simulink model "PMSMdq"  (R2024a)
settings: Solver=ode45  StartTime=0.0  StopTime=10  MaxStep=1  RelTol=1e-3  EnableMultiTasking=on
undefined symbols (not defined in the file or in its folder): Battery, Control, Environment, Motor, Vehicle
libraries: simulink x5, simulink_extras x4, SignalEditorBlockLib x2
settings Model: Creator=Daniel Montesinos  LastModifiedBy=citcea
settings SolverCC: AlgebraicLoopSolver=TrustRegion
settings DataIOCC: LimitDataPoints=on  SaveFormat=Array  SignalLoggingSaveFormat=ModelDataLogs  ReturnWorkspaceOutputs=off
settings OptimizationCC: ReuseModelBlockBuffer=off  ExpressionDepthLimit=2147483647  LifeSpan=inf
settings DebuggingCC: UnderspecifiedInitializationDetection=Classic  MergeDetectMultiDrivingBlocksExec=none  SolverPrmCheckMsg=warning  FcnCallInpInsideContextMsg=warning  UnconnectedInputMsg=warning  UnconnectedOutputMsg=warning  UnconnectedLineMsg=warning  AllowSymbolicDim=off  StateNameClashWarn=warning  SFUnexpectedBacktrackingDiag=warning  SFNoUnconditionalDefaultTransitionDiag=warning  SFExecutionAtInitializationDiag=none  ArithmeticOperatorsInVariantConditions=warning
settings HardwareCC: ProdBitPerPointer=32  ProdBitPerSizeT=32  ProdBitPerPtrDiffT=32  ProdLargestAtomicFloat=None  ProdIntDivRoundTo=Undefined  ProdEndianess=Unspecified  ProdWordSize=32  ProdHWDeviceType=32-bit Generic
settings ModelReferenceCC: EnableRefExpFcnMdlSchedulingChecks=on  PropagateSignalLabelsOutOfModel=off
settings SFSimCC: SimUseLocalCustomCode=off  CustomCodeUndefinedFunction=UseInterfaceOnly
settings RTWCC: RTWUseLocalCustomCode=off  GPUComputeCapability=3.5  DLArmComputeVersion=19.05
settings CodeAppCC: StateflowObjectComments=on
settings GRTTargetCC: TargetLangStandard=C89/C90 (ANSI)  CombineOutputUpdateFcns=off  GRTInterface=on
settings ConfigComp: CovMetricSettings=dw  CovSaveCumulativeToWorkspaceVar=on  CovSaveSingleToWorkspaceVar=on  CovExternalEMLEnable=off  CovSFcnEnable=off

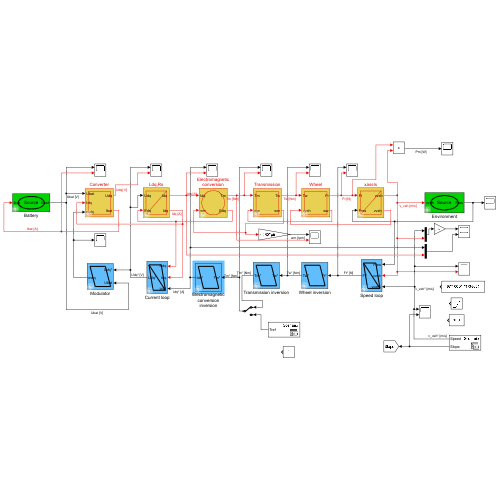
[thumbnail: Simulink's stored preview of the top-level diagram]
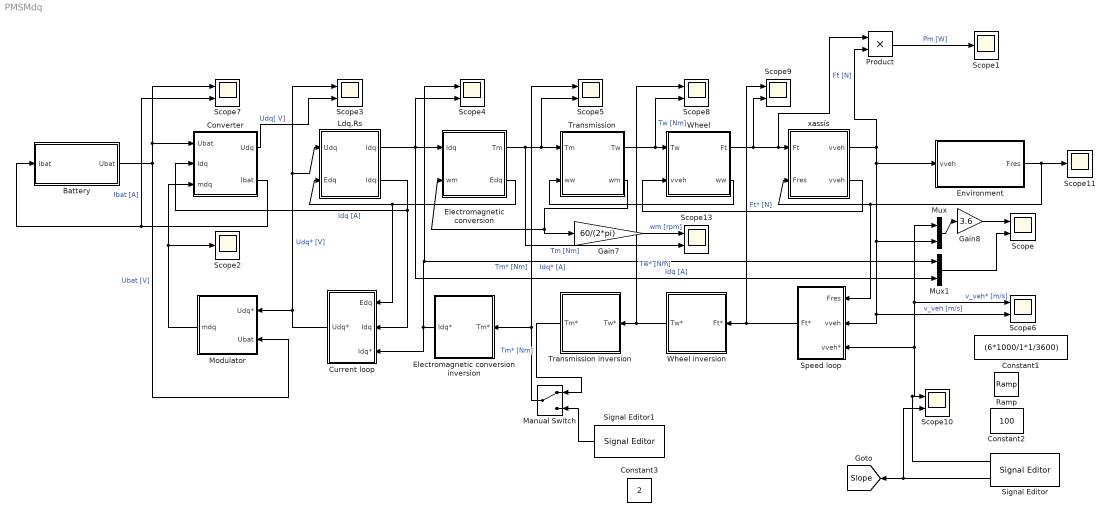
== system PMSMdq ==
  Battery : Subsystem  AncestorBlock=simulink/REM/SE
      mask Display:
      | plot(0,0,100,100, 1.2*[50,57.68,60.77,63.08,64.97,66.58,68,69.26,70.4, 	71.42,72.36,78.28,80,78.28,72.36,71.42,70.4, 	69.26,68,66.58,64.97,63.08,60.77,57.68,50,42.32, 	39.23,36.92,35.03,33.42,32,30.74,29.6,28.58, 	27.64,21.72,20,21.72,27.64,28.58,29.6,30.74,32, 	33.42,35.03,36.92,39.23,42.32,50]-10, 1.2*[20,21,22,23,24,25,26,27,28,29,30,40,50,60,70,71,72, 	73,74,75,76,77,78,79,80,79,78,77,76,75,74,73,72, 	71,70,60,50,40,30,29,28,27,26,25,24,23,22,21,20]-10)
      | disp('Source')
  Constant1 : Constant  Value=(6*1000/1*1/3600)
  Constant2 : Constant  Value=100
  Constant3 : Constant  Value=2
  Converter : Subsystem  AncestorBlock=simulink/REM/EC Elec  mask(Hacheur){}
      mask Display: plot(0,0,100,100,[10,10,90,90,10],[90,10,10,90,90])
  Current loop : Subsystem  AncestorBlock=simulink/SMC/Asservissement Correcteur IP
      mask Display: plot(0,0,100,100, [10,30,90,70,10,90],[90,10,10,90,90,10])
  Electromagnetic conversion : Subsystem  AncestorBlock=simulink/REM/EC EM
      mask Display: plot(0,0,100,100, 1.4*[50,57.68,60.77,63.08,64.97,66.58,68,69.26,70.4, 	71.42,72.36,78.28,80,78.28,72.36,71.42,70.4, 	69.26,68,66.58,64.97,63.08,60.77,57.68,50,42.32, 	39.23,36.92,35.03,33.42,32,30.74,29.6,28.58, 	27.64,21.72,20,21.72,27.64,28.58,29.6,30.74,32, 	33.42,35.03,36.92,39.23,42.32,50]-20, 1.4*[20,21,22,23,24,25,26,27,28,29,30,40,50,60,70,71,72, 	73,74,75,76,77,78,79,80,79,78,77,76,75,74,73,72, 	71,70,60,50,40,30,29,28,27,26,25,24,23,22,21,20]-20)
  Electromagnetic conversion inversion : Subsystem  AncestorBlock=simulink/SMC/Inversion EC avec mesure
      mask Display: plot(0,0,100,100,[10,30,90,70,10],[90,10,10,90,90])
  Environment : Subsystem  AncestorBlock=simulink/REM/SE
      mask Display:
      | plot(0,0,100,100, 1.2*[50,57.68,60.77,63.08,64.97,66.58,68,69.26,70.4, 	71.42,72.36,78.28,80,78.28,72.36,71.42,70.4, 	69.26,68,66.58,64.97,63.08,60.77,57.68,50,42.32, 	39.23,36.92,35.03,33.42,32,30.74,29.6,28.58, 	27.64,21.72,20,21.72,27.64,28.58,29.6,30.74,32, 	33.42,35.03,36.92,39.23,42.32,50]-10, 1.2*[20,21,22,23,24,25,26,27,28,29,30,40,50,60,70,71,72, 	73,74,75,76,77,78,79,80,79,78,77,76,75,74,73,72, 	71,70,60,50,40,30,29,28,27,26,25,24,23,22,21,20]-10)
      | disp('Source')
  Gain7 : Gain  Gain=60/(2*pi)
  Gain8 : Gain  Gain=3.6
  Ldq,Rs : Subsystem  AncestorBlock=simulink/REM/EA  mask(CM){}
      mask Display: plot(0,0,100,100,[10,10,90,90,10],[90,10,10,90,90], [10,90],[10,90])
  Manual Switch : ManualSwitch
  Modulator : Subsystem  AncestorBlock=simulink/SMC/Inversion EC avec mesure
      mask Display: plot(0,0,100,100,[10,30,90,70,10],[90,10,10,90,90])
  Mux : Mux  Inputs=2
  Mux1 : Mux  Inputs=2
  Product : Product
  Ramp : simulink/Sources/Ramp  slope=(3*1000/1*1/3600)/2  start=0  InitialOutput=0
  Scope{,3..10,13} (10 alike) : Scope  NumInputPorts=2
  Scope1 : Scope
  Scope11 : Scope
  Scope2 : Scope
  Signal Editor : SignalEditorBlockLib/Signal Editor  FileName=SpeedRef.mat  ActiveScenario=Scenario  ActiveSignal=Speed  IsBus=off  OutputBusObjectStr=Bus: BusObject  SampleTime=0  Interpolate=off  ZeroCross=off  OutputAfterFinalValue=Setting to zero  Unit=inherit  PreserveSignalName=on  ApplySigPropsToAllScenarios=on  ApplySigPropsToAllSignals=off
  Signal Editor1 : SignalEditorBlockLib/Signal Editor  FileName=Tref.mat  ActiveScenario=Scenario  ActiveSignal=Tref  IsBus=off  OutputBusObjectStr=Bus: BusObject  SampleTime=0  Interpolate=off  ZeroCross=off  OutputAfterFinalValue=Setting to zero  Unit=inherit  PreserveSignalName=on  ApplySigPropsToAllScenarios=on  ApplySigPropsToAllSignals=off
  Speed loop : Subsystem  AncestorBlock=simulink/SMC/Asservissement Correcteur IP
      mask Display: plot(0,0,100,100, [10,30,90,70,10,90],[90,10,10,90,90,10])
  Transmission : Subsystem  AncestorBlock=simulink/REM/EC Elec  mask(Hacheur){}
      mask Display: plot(0,0,100,100,[10,10,90,90,10],[90,10,10,90,90])
  Transmission inversion : Subsystem  AncestorBlock=simulink/SMC/Inversion EC avec mesure
      mask Display: plot(0,0,100,100,[10,30,90,70,10],[90,10,10,90,90])
  Wheel : Subsystem  AncestorBlock=simulink/REM/EC Elec  mask(Hacheur){}
      mask Display: plot(0,0,100,100,[10,10,90,90,10],[90,10,10,90,90])
  Wheel inversion : Subsystem  AncestorBlock=simulink/SMC/Inversion EC avec mesure
      mask Display: plot(0,0,100,100,[10,30,90,70,10],[90,10,10,90,90])
  xassís : Subsystem  AncestorBlock=simulink/REM/EA  mask(CM){}
      mask Display: plot(0,0,100,100,[10,10,90,90,10],[90,10,10,90,90], [10,90],[10,90])
  tag scope: Slope=global
  wires:
  xassís/1(vveh) -> Product/2, Environment/1(vveh), Scope6/2, Speed loop/2(vveh), Mux/2  "v_veh [m/s]"
  Environment/1(Fres) -> Scope11/1, Speed loop/1(Fres), xassís/2(Fres)
  Mux/1 -> Gain8/1
  xassís/2("vveh ") -> Wheel/2(vveh)
  Transmission/1(Tw) -> Scope8/2, Wheel/1(Tw)  "Tw [Nm]"
  Wheel/2(ww) -> Transmission/2(ww)
  Wheel inversion/1(Tw*) -> Scope8/1, Transmission inversion/1(Tw*)  "Tw* [Nm]"
  Transmission/2(wm) -> Electromagnetic conversion/2(wm), Gain7/1
  Electromagnetic conversion/1(Tm) -> Scope13/2, Scope5/2, Transmission/1(Tm)  "Tm [Nm]"
  Ldq,Rs/1("Idq ") -> Scope4/2, Electromagnetic conversion/1(Idq), Mux1/2  "Idq [A]"
  Electromagnetic conversion/2(Edq) -> Current loop/1(Edq), Ldq,Rs/2(Edq)
  Electromagnetic conversion inversion/1(Idq*) -> Scope4/1, Mux1/1, Current loop/3(Idq*)  "Idq* [A]"
  Ldq,Rs/2(Idq) -> Current loop/2(Idq), Converter/2(Idq)  "Idq [A]"
  Manual Switch/1 -> Scope5/1, Electromagnetic conversion inversion/1(Tm*)  "Tm* [Nm]"
  Modulator/1(mdq) -> Converter/3(mdq), Scope2/1
  Converter/2(Ibat) -> Battery/1(Ibat), Scope7/2  "Ibat [A]"
  Battery/1(Ubat) -> Modulator/2(Ubat), Converter/1(Ubat), Scope7/1  "Ubat [V]"
  Speed loop/1(Ft*) -> Scope9/1, Wheel inversion/1(Ft*)  "Ft* [N]"
  Wheel/1(Ft) -> Scope9/2, Product/1, xassís/1(Ft)  "Ft [N]"
  Current loop/1(Udq*) -> Ldq,Rs/1(Udq), Scope3/1, Modulator/1(Udq*)  "Udq* [V]"
  Converter/1(Udq) -> Scope3/2  "Udq[ V]"
  Gain7/1 -> Scope13/1  "wm [rpm]"
  Gain8/1 -> Scope/1
  Mux1/1 -> Scope/2
  Signal Editor/1 -> Speed loop/3(vveh*), Scope6/1, Mux/1, Scope10/1  "v_veh* [m/s]"
  Product/1 -> Scope1/1  "Pm [W]"
  Signal Editor/2 -> Scope10/2, [Slope]
  Signal Editor1/1 -> Manual Switch/2
  Transmission inversion/1(Tm*) -> Manual Switch/1  "Tm* [Nm]"

== system PMSMdq/Battery ==
  Ibat : Inport
  Constant : Constant  Value=Battery.Electrical.Ubat
  Terminator : Terminator
  Ubat : Outport  InitialOutput=0  VectorParamsAs1DForOutWhenUnconnected=off
  wires:
  Ibat/1 -> Terminator/1
  Constant/1 -> Ubat/1

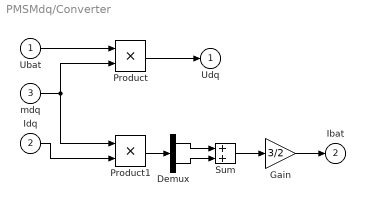
== system PMSMdq/Converter ==
  Ubat : Inport
  Idq : Inport  Port=2
  mdq : Inport  Port=3
  Demux : Demux  Outputs=2
  Gain : Gain  Gain=3/2
  Product : Product
  Product1 : Product
  Sum : Sum
  Udq : Outport  InitialOutput=0  VectorParamsAs1DForOutWhenUnconnected=off
  Ibat : Outport  Port=2  InitialOutput=0  VectorParamsAs1DForOutWhenUnconnected=off
  wires:
  Ubat/1 -> Product/1
  mdq/1 -> Product1/1, Product/2
  Product/1 -> Udq/1
  Product1/1 -> Demux/1
  Demux/1 -> Sum/1
  Demux/2 -> Sum/2
  Sum/1 -> Gain/1
  Gain/1 -> Ibat/1
  Idq/1 -> Product1/2

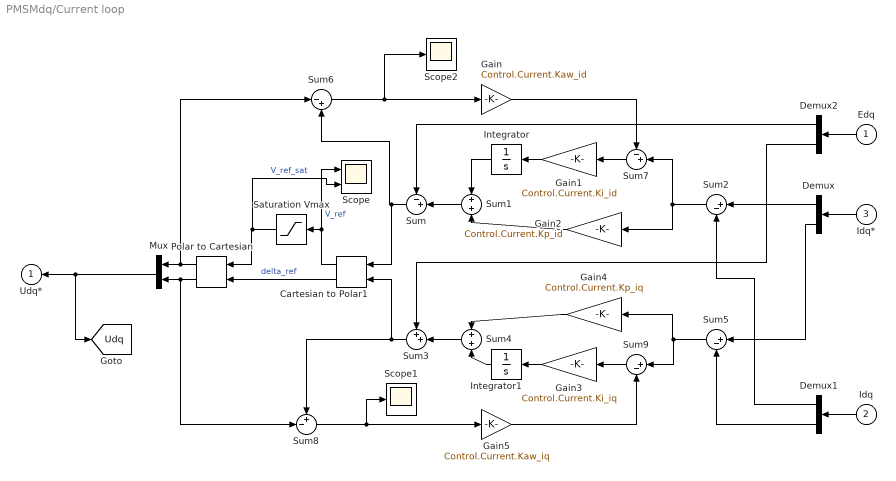
== system PMSMdq/Current loop ==
  Edq : Inport
  Idq : Inport  Port=2
  Idq* : Inport  Port=3
  Cartesian to Polar1 : simulink_extras/Transformations/Cartesian to Polar
  Demux : Demux  Outputs=2
  Demux1 : Demux  Outputs=2
  Demux2 : Demux  Outputs=2
  Gain : Gain  Gain=Control.Current.Kaw_id
  Gain1 : Gain  Gain=Control.Current.Ki_id
  Gain2 : Gain  Gain=Control.Current.Kp_id
  Gain3 : Gain  Gain=Control.Current.Ki_iq
  Gain4 : Gain  Gain=Control.Current.Kp_iq
  Gain5 : Gain  Gain=Control.Current.Kaw_iq
  Integrator : Integrator
  Integrator1 : Integrator
  Mux : Mux  Inputs=2
  Polar to Cartesian : simulink_extras/Transformations/Polar to Cartesian
  Saturation Vmax : Saturate  UpperLimit=Motor.Electrical.Umax  LowerLimit=-Motor.Electrical.Umax
  Scope : Scope  NumInputPorts=2
  Scope1 : Scope
  Scope2 : Scope
  Sum : Sum  Inputs=-+|
  Sum1 : Sum
  Sum2 : Sum  Inputs=|+-
  Sum3 : Sum  Inputs=++|
  Sum4 : Sum
  Sum5 : Sum  Inputs=|+-
  Sum6 : Sum  Inputs=|-+
  Sum7 : Sum  Inputs=-+|
  Sum8 : Sum  Inputs=+-|
  Sum9 : Sum  Inputs=|+-
  Udq* : Outport  InitialOutput=0  VectorParamsAs1DForOutWhenUnconnected=off
  tag scope: Udq=global
  wires:
  Sum1/1 -> Sum/2
  Gain1/1 -> Integrator/1
  Sum2/1 -> Sum7/2, Gain2/1
  Integrator1/1 -> Sum4/2
  Gain3/1 -> Integrator1/1
  Gain4/1 -> Sum4/1
  Sum5/1 -> Sum9/1, Gain4/1
  Sum4/1 -> Sum3/2
  Idq*/1 -> Demux/1
  Demux/1 -> Sum2/1
  Demux/2 -> Sum5/1
  Idq/1 -> Demux1/1
  Demux1/1 -> Sum2/2
  Demux1/2 -> Sum5/2
  Edq/1 -> Demux2/1
  Demux2/2 -> Sum3/1
  Mux/1 -> [Udq], Udq*/1
  Demux2/1 -> Sum/1
  Cartesian to Polar1/1 -> Scope/1, Saturation Vmax/1  "V_ref"
  Saturation Vmax/1 -> Scope/2, Polar to Cartesian/1  "V_ref_sat"
  Cartesian to Polar1/2 -> Polar to Cartesian/2  "delta_ref"
  Sum/1 -> Sum6/2, Cartesian to Polar1/1
  Sum3/1 -> Sum8/1, Cartesian to Polar1/2
  Polar to Cartesian/1 -> Sum6/1, Mux/1
  Polar to Cartesian/2 -> Sum8/2, Mux/2
  Integrator/1 -> Sum1/1
  Gain2/1 -> Sum1/2
  Sum7/1 -> Gain1/1
  Sum6/1 -> Scope2/1, Gain/1
  Gain/1 -> Sum7/1
  Sum9/1 -> Gain3/1
  Sum8/1 -> Scope1/1, Gain5/1
  Gain5/1 -> Sum9/2

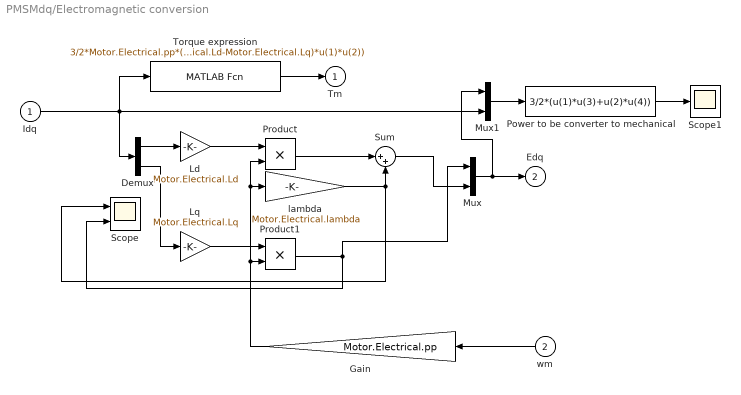
== system PMSMdq/Electromagnetic conversion ==
  Idq : Inport
  wm : Inport  Port=2
  Demux : Demux  Outputs=2
  Gain : Gain  Gain=Motor.Electrical.pp
  Ld : Gain  Gain=Motor.Electrical.Ld
  Lq : Gain  Gain=Motor.Electrical.Lq
  Mux : Mux  Inputs=2
  Mux1 : Mux  Inputs=2
  Power to be converter to mechanical : MATLABFcn  MATLABFcn=3/2*(u(1)*u(3)+u(2)*u(4))
  Product : Product
  Product1 : Product
  Scope : Scope  NumInputPorts=2
  Scope1 : Scope
  Sum : Sum  Inputs=|++
  Torque expression : MATLABFcn  MATLABFcn=3/2*Motor.Electrical.pp*(Motor.Electrical.lambda*u(2)+(Motor.Electrical.Ld-Motor.Electrical.Lq)*u(1)*u(2))  OutputDimensions=1
  lambda : Gain  Gain=Motor.Electrical.lambda
  Tm : Outport  InitialOutput=0  VectorParamsAs1DForOutWhenUnconnected=off
  Edq : Outport  Port=2  InitialOutput=0  VectorParamsAs1DForOutWhenUnconnected=off
  wires:
  Torque expression/1 -> Tm/1
  Idq/1 -> Demux/1, Torque expression/1, Mux1/2
  Demux/1 -> Ld/1
  Demux/2 -> Lq/1
  Ld/1 -> Product/1
  wm/1 -> Gain/1
  Lq/1 -> Product1/1
  Product/1 -> Sum/1
  lambda/1 -> Scope/1, Sum/2
  Product1/1 -> Scope/2, Mux/1
  Mux/1 -> Mux1/1, Edq/1
  Mux1/1 -> Power to be converter to mechanical/1
  Power to be converter to mechanical/1 -> Scope1/1
  Sum/1 -> Mux/2
  Gain/1 -> Product/2, lambda/1, Product1/2

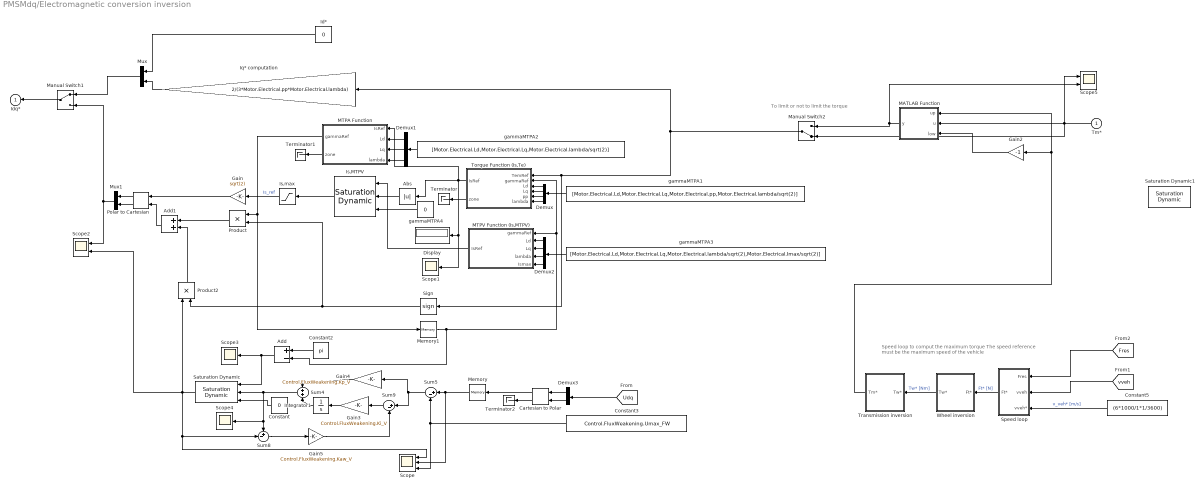
== system PMSMdq/Electromagnetic conversion inversion ==
  note: To limit or not to limit the torque
  note: Speed loop to comput the maximum torque
      | The speed reference must be the maximum speed of the vehicle
  Tm* : Inport
  Abs : Abs  SaturateOnIntegerOverflow=off
  Add : Sum  Inputs=+-
  Add1 : Sum
  Cartesian to Polar : simulink_extras/Transformations/Cartesian to Polar
  Constant : Constant  Value=0
  Constant2 : Constant  Value=pi
  Constant3 : Constant  Value=Control.FluxWeakening.Umax_FW  SampleTime=-1
  Constant5 : Constant  Value=(6*1000/1*1/3600)
  Demux : Demux
  Demux1 : Demux  Outputs=3
  Demux2 : Demux
  Demux3 : Demux  Outputs=2
  Display : Display
  Gain : Gain  Gain=sqrt(2)
  Gain2 : Gain  Gain=-1
  Gain3 : Gain  Gain=Control.FluxWeakening.Ki_V
  Gain4 : Gain  Gain=Control.FluxWeakening.Kp_V
  Gain5 : Gain  Gain=Control.FluxWeakening.Kaw_V
  Id* : Constant  Value=0
  Integrator1 : Integrator
  Iq* computation : Gain  Gain=2/(3*Motor.Electrical.pp*Motor.Electrical.lambda)
  Is,MTPV : simulink/Discontinuities/Saturation Dynamic  OutMin=[]  OutMax=[]  OutDataTypeStr=Inherit: Same as second input  OutDataType=fixdt(1, 16)  OutScaling=2^-10  DoSatur=off
  Is,max : Saturate  UpperLimit=Motor.Electrical.Imax  LowerLimit=0
  MATLAB Function : MATLAB Function  TreatAsAtomicUnit=on
  MTPA Function : MATLAB Function  TreatAsAtomicUnit=on
  MTPV Function (Is,MTPV) : MATLAB Function  TreatAsAtomicUnit=on
  Manual Switch1 : ManualSwitch
  Manual Switch2 : ManualSwitch  CurrentSetting=0
  Memory : Memory
  Memory1 : Memory  InitialCondition=pi/2
  Mux : Mux  Inputs=2
  Mux1 : Mux  Inputs=2
  Polar to Cartesian : simulink_extras/Transformations/Polar to Cartesian
  Product : Product
  Product2 : Product
  Saturation Dynamic : simulink/Discontinuities/Saturation Dynamic  OutMin=[]  OutMax=[]  OutDataTypeStr=Inherit: Same as second input  OutDataType=fixdt(1, 16)  OutScaling=2^-10  DoSatur=off
  Saturation Dynamic1 : simulink/Discontinuities/Saturation Dynamic  OutMin=[]  OutMax=[]  OutDataTypeStr=Inherit: Same as second input  OutDataType=fixdt(1, 16)  OutScaling=2^-10  DoSatur=off
  Scope : Scope  NumInputPorts=3
  Scope1 : Scope
  Scope2 : Scope  NumInputPorts=2
  Scope3 : Scope
  Scope4 : Scope
  Scope5 : Scope  NumInputPorts=2
  Sign : Signum
  Speed loop : Subsystem  AncestorBlock=simulink/SMC/Asservissement Correcteur IP
      mask Display: plot(0,0,100,100, [10,30,90,70,10,90],[90,10,10,90,90,10])
  Sum4 : Sum
  Sum5 : Sum  Inputs=|+-
  Sum8 : Sum  Inputs=+-|
  Sum9 : Sum  Inputs=|+-
  Terminator : Terminator
  Terminator1 : Terminator
  Terminator2 : Terminator
  Torque Function (Is,Te) : MATLAB Function  TreatAsAtomicUnit=on
  Transmission inversion : Subsystem  AncestorBlock=simulink/SMC/Inversion EC avec mesure
      mask Display: plot(0,0,100,100,[10,30,90,70,10],[90,10,10,90,90])
  Wheel inversion : Subsystem  AncestorBlock=simulink/SMC/Inversion EC avec mesure
      mask Display: plot(0,0,100,100,[10,30,90,70,10],[90,10,10,90,90])
  gammaMTPA1 : Constant  Value=[Motor.Electrical.Ld,Motor.Electrical.Lq,Motor.Electrical.pp,Motor.Electrical.lambda/sqrt(2)]  SampleTime=-1
  gammaMTPA2 : Constant  Value=[Motor.Electrical.Ld,Motor.Electrical.Lq,Motor.Electrical.lambda/sqrt(2)]  SampleTime=-1
  gammaMTPA3 : Constant  Value=[Motor.Electrical.Ld,Motor.Electrical.Lq,Motor.Electrical.lambda/sqrt(2),Motor.Electrical.Imax/sqrt(2)]  SampleTime=-1
  gammaMTPA4 : Constant  Value=0  SampleTime=-1
  Idq* : Outport  InitialOutput=0  VectorParamsAs1DForOutWhenUnconnected=off
  wires:
  MATLAB Function/1(y) -> Scope5/2, Manual Switch2/1
  gammaMTPA1/1 -> Demux/1
  Demux1/1 -> MTPA Function/2(Ld)
  Torque Function (Is,Te)/1(IsRef) -> Scope1/1, Display/1, Abs/1, MTPA Function/1(IsRef)
  MTPV Function (Is,MTPV)/1(IsRef) -> Is,MTPV/1
  gammaMTPA2/1 -> Demux1/1
  Demux2/2 -> MTPV Function (Is,MTPV)/3(Lq)
  Demux/1 -> Torque Function (Is,Te)/3(Ld)
  Demux1/3 -> MTPA Function/4(lambda)
  Demux2/4 -> MTPV Function (Is,MTPV)/5(Ismax)
  Demux/3 -> Torque Function (Is,Te)/5(pp)
  Demux/4 -> Torque Function (Is,Te)/6(lambda)
  Demux/2 -> Torque Function (Is,Te)/4(Lq)
  gammaMTPA3/1 -> Demux2/1
  MTPA Function/2(zone) -> Terminator1/1
  Is,MTPV/1 -> Is,max/1
  Torque Function (Is,Te)/2(zone) -> Terminator/1
  Demux1/2 -> MTPA Function/3(Lq)
  gammaMTPA4/1 -> Is,MTPV/3
  Demux2/3 -> MTPV Function (Is,MTPV)/4(lambda)
  Demux2/1 -> MTPV Function (Is,MTPV)/2(Ld)
  Is,max/1 -> Gain/1  "Is_ref"
  MTPA Function/1(gammaRef) -> Memory1/1, Product/1
  Memory1/1 -> Add/2, MTPV Function (Is,MTPV)/1(gammaRef), Torque Function (Is,Te)/2(gammaRef)
  Polar to Cartesian/1 -> Mux1/1
  Polar to Cartesian/2 -> Mux1/2
  Mux1/1 -> Scope2/1, Manual Switch1/2
  Gain/1 -> Polar to Cartesian/1
  Abs/1 -> Is,MTPV/2
  Sign/1 -> Product2/2, Product/2
  Demux3/2 -> Cartesian to Polar/2
  Demux3/1 -> Cartesian to Polar/1
  [Udq] -> Demux3/1
  Gain5/1 -> Sum9/2
  Cartesian to Polar/1 -> Memory/1
  Sum5/1 -> Gain4/1, Sum9/1
  Sum4/1 -> Scope4/1, Sum8/1, Saturation Dynamic/2
  Gain3/1 -> Integrator1/1
  Gain4/1 -> Sum4/1
  Constant3/1 -> Sum5/2, Scope/3
  Sum9/1 -> Gain3/1
  Integrator1/1 -> Sum4/2
  Cartesian to Polar/2 -> Terminator2/1
  Constant/1 -> Saturation Dynamic/3
  Add/1 -> Scope3/1, Saturation Dynamic/1
  Constant2/1 -> Add/1
  Sum8/1 -> Gain5/1
  Saturation Dynamic/1 -> Scope/1, Sum8/2, Scope2/2, Product2/1
  Product/1 -> Add1/1
  Add1/1 -> Polar to Cartesian/2
  Product2/1 -> Add1/2
  Memory/1 -> Scope/2, Sum5/1
  Manual Switch1/1 -> Idq*/1
  Mux/1 -> Manual Switch1/1
  Iq* computation/1 -> Mux/2
  Id*/1 -> Mux/1
  Transmission inversion/1(Tm*) -> MATLAB Function/1(up), Gain2/1
  Gain2/1 -> MATLAB Function/3(low)
  Tm*/1 -> MATLAB Function/2(u), Manual Switch2/2, Scope5/1
  Manual Switch2/1 -> Iq* computation/1, Sign/1, Torque Function (Is,Te)/1(TemRef)
  Constant5/1 -> Speed loop/3(vveh*)  "v_veh* [m/s]"
  Speed loop/1(Ft*) -> Wheel inversion/1(Ft*)  "Ft* [N]"
  Wheel inversion/1(Tw*) -> Transmission inversion/1(Tw*)  "Tw* [Nm]"
  [vveh] -> Speed loop/2(vveh)
  [Fres] -> Speed loop/1(Fres)

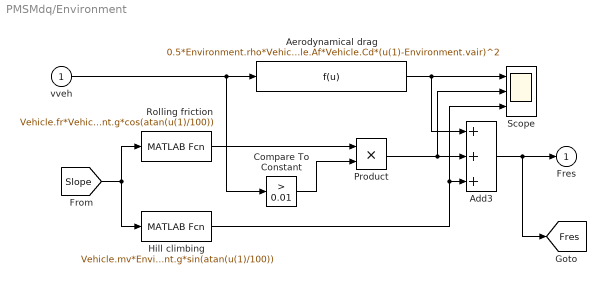
== system PMSMdq/Environment ==
  vveh : Inport
  Add3 : Sum  Inputs=+++
  Aerodynamical drag : Fcn  Expr=0.5*Environment.rho*Vehicle.Af*Vehicle.Cd*(u(1)-Environment.vair)^2
  Compare To Constant : simulink/Logic and Bit Operations/Compare To Constant  relop=>  const=0.01  OutDataTypeStr=boolean  ZeroCross=off
  Hill climbing : MATLABFcn  MATLABFcn=Vehicle.mv*Environment.g*sin(atan(u(1)/100))
  Product : Product
  Rolling friction : MATLABFcn  MATLABFcn=Vehicle.fr*Vehicle.mv*Environment.g*cos(atan(u(1)/100))
  Scope : Scope  NumInputPorts=3
  Fres : Outport  InitialOutput=0  VectorParamsAs1DForOutWhenUnconnected=off
  tag scope: Fres=global
  wires:
  Aerodynamical drag/1 -> Scope/1, Add3/1
  Hill climbing/1 -> Scope/3, Add3/3
  Product/1 -> Scope/2, Add3/2
  Add3/1 -> [Fres], Fres/1
  vveh/1 -> Compare To Constant/1, Aerodynamical drag/1
  Compare To Constant/1 -> Product/2
  Rolling friction/1 -> Product/1
  [Slope] -> Hill climbing/1, Rolling friction/1

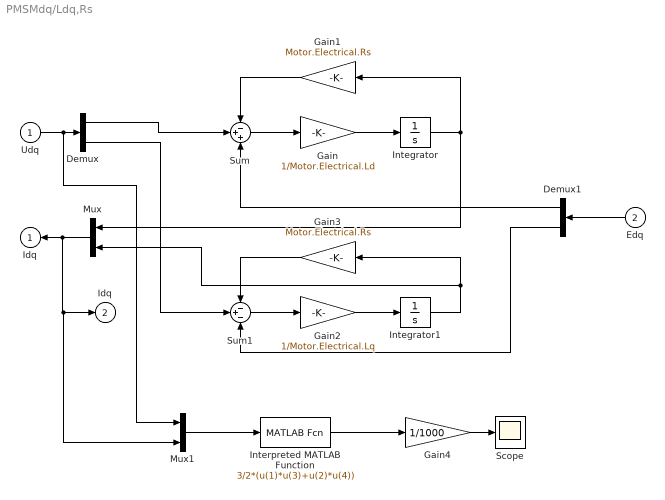
== system PMSMdq/Ldq,Rs ==
  Udq : Inport
  Edq : Inport  Port=2
  Demux : Demux  Outputs=2
  Demux1 : Demux  Outputs=2
  Gain : Gain  Gain=1/Motor.Electrical.Ld
  Gain1 : Gain  Gain=Motor.Electrical.Rs
  Gain2 : Gain  Gain=1/Motor.Electrical.Lq
  Gain3 : Gain  Gain=Motor.Electrical.Rs
  Gain4 : Gain  Gain=1/1000
  Integrator : Integrator
  Integrator1 : Integrator
  Interpreted MATLAB Function : MATLABFcn  MATLABFcn=3/2*(u(1)*u(3)+u(2)*u(4))
  Mux : Mux  Inputs=2
  Mux1 : Mux  Inputs=2
  Scope : Scope
  Sum : Sum  Inputs=-++
  Sum1 : Sum  Inputs=-+-
  "Idq " : Outport  InitialOutput=0  VectorParamsAs1DForOutWhenUnconnected=off
  Idq : Outport  Port=2  InitialOutput=0  VectorParamsAs1DForOutWhenUnconnected=off
  wires:
  Integrator/1 -> Mux/1, Gain1/1
  Gain/1 -> Integrator/1
  Sum/1 -> Gain/1
  Gain1/1 -> Sum/1
  Gain3/1 -> Sum1/1
  Gain2/1 -> Integrator1/1
  Integrator1/1 -> Gain3/1, Mux/2
  Sum1/1 -> Gain2/1
  Udq/1 -> Mux1/1, Demux/1
  Demux/1 -> Sum/2
  Demux/2 -> Sum1/2
  Mux/1 -> Mux1/2, Idq/1, "Idq "/1
  Edq/1 -> Demux1/1
  Mux1/1 -> Interpreted MATLAB Function/1
  Interpreted MATLAB Function/1 -> Gain4/1
  Gain4/1 -> Scope/1
  Demux1/1 -> Sum/3
  Demux1/2 -> Sum1/3

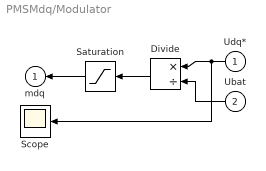
== system PMSMdq/Modulator ==
  Udq* : Inport
  Ubat : Inport  Port=2
  Divide : Product  Inputs=*/
  Saturation : Saturate  UpperLimit=1  LowerLimit=-1
  Scope : Scope
  mdq : Outport  InitialOutput=0  VectorParamsAs1DForOutWhenUnconnected=off
  wires:
  Udq*/1 -> Scope/1, Divide/1
  Ubat/1 -> Divide/2
  Divide/1 -> Saturation/1
  Saturation/1 -> mdq/1

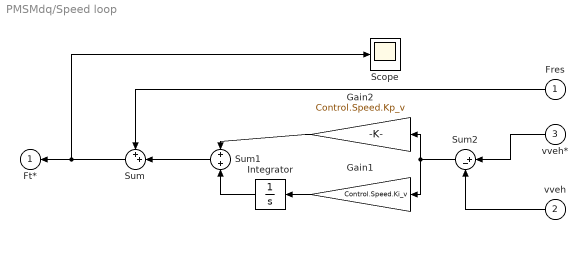
== system PMSMdq/Speed loop ==
  Fres : Inport
  vveh : Inport  Port=2
  vveh* : Inport  Port=3
  Gain1 : Gain  Gain=Control.Speed.Ki_v
  Gain2 : Gain  Gain=Control.Speed.Kp_v
  Integrator : Integrator
  Scope : Scope
  Sum : Sum  Inputs=++|
  Sum1 : Sum
  Sum2 : Sum  Inputs=|+-
  Ft* : Outport  InitialOutput=0  VectorParamsAs1DForOutWhenUnconnected=off
  wires:
  Sum/1 -> Scope/1, Ft*/1
  Fres/1 -> Sum/1
  Gain1/1 -> Integrator/1
  Integrator/1 -> Sum1/2
  Gain2/1 -> Sum1/1
  Sum1/1 -> Sum/2
  vveh*/1 -> Sum2/1
  vveh/1 -> Sum2/2
  Sum2/1 -> Gain2/1, Gain1/1

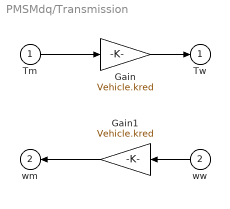
== system PMSMdq/Transmission ==
  Tm : Inport
  ww : Inport  Port=2
  Gain : Gain  Gain=Vehicle.kred
  Gain1 : Gain  Gain=Vehicle.kred
  Tw : Outport  InitialOutput=0  VectorParamsAs1DForOutWhenUnconnected=off
  wm : Outport  Port=2  InitialOutput=0  VectorParamsAs1DForOutWhenUnconnected=off
  wires:
  Tm/1 -> Gain/1
  Gain/1 -> Tw/1
  Gain1/1 -> wm/1
  ww/1 -> Gain1/1

== system PMSMdq/Transmission inversion ==
  Tw* : Inport
  Gain : Gain  Gain=1/Vehicle.kred
  Tm* : Outport  InitialOutput=0  VectorParamsAs1DForOutWhenUnconnected=off
  wires:
  Tw*/1 -> Gain/1
  Gain/1 -> Tm*/1

== system PMSMdq/Wheel ==
  Tw : Inport
  vveh : Inport  Port=2
  Gain : Gain  Gain=1/Vehicle.rw
  Gain1 : Gain  Gain=1/Vehicle.rw
  Ft : Outport  InitialOutput=0  VectorParamsAs1DForOutWhenUnconnected=off
  ww : Outport  Port=2  InitialOutput=0  VectorParamsAs1DForOutWhenUnconnected=off
  wires:
  Tw/1 -> Gain/1
  Gain/1 -> Ft/1
  Gain1/1 -> ww/1
  vveh/1 -> Gain1/1

== system PMSMdq/Wheel inversion ==
  Ft* : Inport
  Gain : Gain  Gain=Vehicle.rw
  Tw* : Outport  InitialOutput=0  VectorParamsAs1DForOutWhenUnconnected=off
  wires:
  Gain/1 -> Tw*/1
  Ft*/1 -> Gain/1

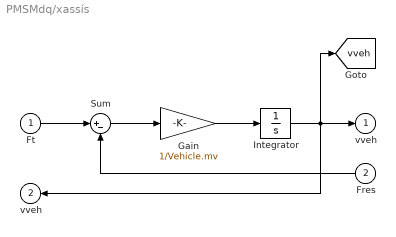
== system PMSMdq/xassís ==
  Ft : Inport
  Fres : Inport  Port=2
  Gain : Gain  Gain=1/Vehicle.mv
  Integrator : Integrator
  Sum : Sum  Inputs=|+-
  vveh : Outport  InitialOutput=0  VectorParamsAs1DForOutWhenUnconnected=off
  "vveh " : Outport  Port=2  InitialOutput=0  VectorParamsAs1DForOutWhenUnconnected=off
  tag scope: vveh=global
  wires:
  Ft/1 -> Sum/1
  Fres/1 -> Sum/2
  Sum/1 -> Gain/1
  Gain/1 -> Integrator/1
  Integrator/1 -> [vveh], vveh/1, "vveh "/1

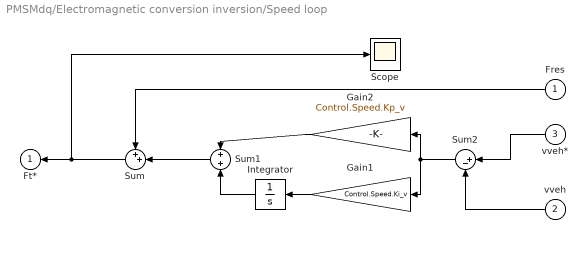
== system PMSMdq/Electromagnetic conversion inversion/Speed loop ==
  Fres : Inport
  vveh : Inport  Port=2
  vveh* : Inport  Port=3
  Gain1 : Gain  Gain=Control.Speed.Ki_v
  Gain2 : Gain  Gain=Control.Speed.Kp_v
  Integrator : Integrator
  Scope : Scope
  Sum : Sum  Inputs=++|
  Sum1 : Sum
  Sum2 : Sum  Inputs=|+-
  Ft* : Outport  InitialOutput=0  VectorParamsAs1DForOutWhenUnconnected=off
  wires:
  Sum/1 -> Scope/1, Ft*/1
  Fres/1 -> Sum/1
  Gain1/1 -> Integrator/1
  Integrator/1 -> Sum1/2
  Gain2/1 -> Sum1/1
  Sum1/1 -> Sum/2
  vveh*/1 -> Sum2/1
  vveh/1 -> Sum2/2
  Sum2/1 -> Gain2/1, Gain1/1

== system PMSMdq/Electromagnetic conversion inversion/Transmission inversion ==
  Tw* : Inport
  Gain : Gain  Gain=1/Vehicle.kred
  Tm* : Outport  InitialOutput=0  VectorParamsAs1DForOutWhenUnconnected=off
  wires:
  Tw*/1 -> Gain/1
  Gain/1 -> Tm*/1

== system PMSMdq/Electromagnetic conversion inversion/Wheel inversion ==
  Ft* : Inport
  Gain : Gain  Gain=Vehicle.rw
  Tw* : Outport  InitialOutput=0  VectorParamsAs1DForOutWhenUnconnected=off
  wires:
  Gain/1 -> Tw*/1
  Ft*/1 -> Gain/1

== matlab function PMSMdq/Electromagnetic conversion inversion/MTPA Function ==
  data: IsRef input; gammaRef output; Ld input; Lq input; lambda input; zone output
function [gammaRef,zone] = fcn(IsRef,Ld,Lq,lambda)
% This function calculates the gammaRef from the MTPA condition for SPMSMs
% and IPMSMs.
% Inputs:
%   IsRef: Reference modulus current (A)
%   Ld: d-axis inductance (H)
%   Lq: q-axis inductance (H)
%   lambda: flux-linkage (V·s/rad)

% Outputs:
%   gammaRef: Reference angle current (rad)
%   gammaRef = acos(((beta/IsRef) - sqrt(beta^2/IsRef^2 + 8)) / 4);

    beta = lambda / (Lq-Ld);

    if (IsRef <= 0)
        gammaRef = pi / 2;
        zone = 1;
    else
        gammaRef = sqrt(beta*beta/(IsRef*IsRef) + 8);
        gammaRef = (beta / IsRef - gammaRef) / 4;
        if (gammaRef >= 0)
            gammaRef = pi / 2;
            zone = 2;
        else
            gammaRef = acos(gammaRef);
            zone = 3;
        end
    end
return

== matlab function PMSMdq/Electromagnetic conversion inversion/MTPV Function (Is,MTPV) ==
  data: gammaRef input; IsRef output; Ld input; Lq input; lambda input; Ismax input
function IsRef = fcn(gammaRef,Ld,Lq,lambda,Ismax)
% This function calculates the modulus current from the MTPV condition for SPMSMs
% and IPMSMs.
% Inputs:
%   gammaRef: Reference angle current (rad)
%   Ld: d-axis inductance (H)
%   Lq: q-axis inductance (H)
%   lambda: flux-linkage (V·s/rad)
%   Ismax: Maximum stator current (A)

% Outputs:
%   IsRef: Reference modulus current (A)

    xi = Lq / Ld;
    Isc = lambda / Ld;
    beta = lambda/(Lq-Ld);
    mu = beta - lambda/Ld;

    if (Ld == Lq)   % SPMSMs
        IsRef = abs (lambda / Ld / cos(gammaRef));
    else            % IPMSMs
        aux_MTPV = cos(gammaRef)^2 - xi^2*sin(gammaRef)^2;
        IsRef = aux_MTPV * (mu^2 - xi^2*beta^2);
        IsRef = mu^2*cos(gammaRef)^2 - IsRef;
        if (IsRef < 0)
            IsRef = max(Ismax,Isc);
        else
            IsRef = mu*cos(gammaRef) + sqrt(IsRef);
            IsRef = IsRef / (2 * aux_MTPV);
        end
%         IsRef = abs (Ismax / cos(gammaRef));
    end

return

== matlab function PMSMdq/Electromagnetic conversion inversion/MATLAB Function ==
  data: up input; y output; u input; low input
function y   = fcn(up,u,low)

if u>=up
    y=up;
elseif u<=low
    y=low;
else
    y=u;
end

== matlab function PMSMdq/Electromagnetic conversion inversion/Torque Function (Is,Te) ==
  data: TemRef input; IsRef output; gammaRef input; Ld input; Lq input; pp input; lambda input; zone output
function [IsRef,zone] = fcn(TemRef,gammaRef,Ld,Lq,pp,lambda)
% This function calculates the modulus current from the previous current angle
% considering the torque set point.
% Inputs:
%   gammaRef: Reference angle current (rad)
%   Ld: d-axis inductance (H)
%   Lq: q-axis inductance (H)
%   pp: pair of poles
%   lambda: flux-linkage (V·s/rad)

% Outputs:
%   IsRef: Reference modulus current (A)

    alpha = 1/(3*pp*(Lq-Ld));
    beta = lambda/(Lq-Ld);

    if (Ld == Lq)   % SPMSM
        IsRef = TemRef/(3*pp*lambda*sin(gammaRef));
        zone = 1;
    else            % IPMSM
        if (gammaRef <= pi/2)
            IsRef = TemRef/(3*pp*lambda*sin(gammaRef));
            zone = 2;
        else
            IsRef = 4 * TemRef * alpha * cos(gammaRef) / sin(gammaRef);
            if ((beta^2 - IsRef) <= 0)
                IsRef = TemRef/(3*pp*lambda*sin(gammaRef));
                zone = 3;
            else
                IsRef = sqrt(beta^2 - IsRef);
                IsRef = (beta - IsRef) / (2 * cos(gammaRef));
                zone = 4;
            end
        end
    end

return
